simulink model "model_i3_c3_f2_equal_h2o"  (Simulink 8.4)
settings: Solver=ode3  StartTime=0.0  StopTime=1  FixedStep=0.0001  RelTol=1e-3
libraries: powerlib x28
settings Model: Creator=yh3wong  LastModifiedBy=yh3wong
settings DataIOCC: LimitDataPoints=off  SignalLoggingSaveFormat=Dataset  SaveOutput=off  SaveTime=off
settings OptimizationCC: ExpressionDepthLimit=128
settings DebuggingCC: UnderspecifiedInitializationDetection=Simplified  MergeDetectMultiDrivingBlocksExec=error  FcnCallInpInsideContextMsg=EnableAllAsError  UnconnectedInputMsg=none  UnconnectedOutputMsg=none  UnconnectedLineMsg=none  StateNameClashWarn=none
settings GRTTargetCC: CombineOutputUpdateFcns=on  GRTInterface=off

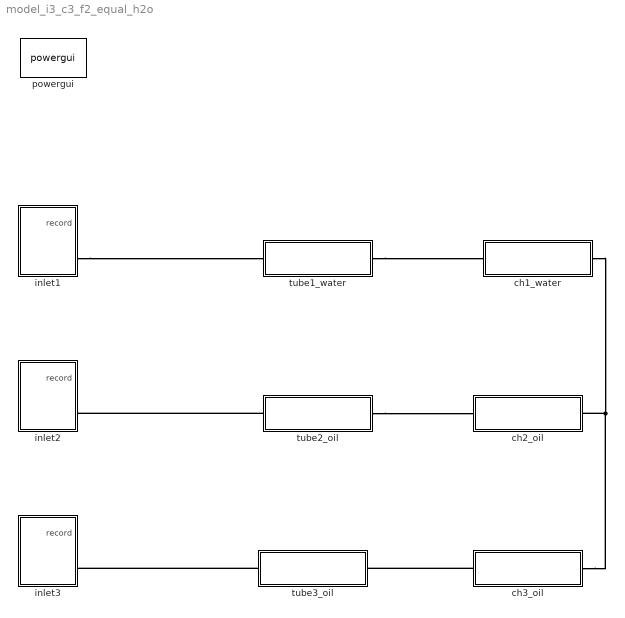
== system model_i3_c3_f2_equal_h2o ==
  ch1_water : Subsystem
  ch2_oil : Subsystem
  ch3_oil : Subsystem
  inlet1 : Subsystem
  inlet2 : Subsystem
  inlet3 : Subsystem
  powergui : powerlib/powergui  Priority=1  SimulationMode=Continuous  SolverType=Tustin/Backward Euler (TBE)  SampleTime=0.1  frequency=60  SPID=off  DisableSnubberDevices=off  DisableRonSwitches=off  DisableVfSwitches=off  SwTol=0  DisplayEquations=off  Interpol=off  methode=off  Ts=100  frequencyindice=0  Pbase=100e6  ErrMax=1e-4  Iterations=50  UnitsV=kV  UnitsW=MW  FunctionMessages=off  echomessages=off  HookPort=off  EnableUseOfTLC=off  x0status=blocks  RestoreLinks=warning  ResistiveCurrentMeasurement=off  Frange=[0:2:500]  Ylog=off  Xlog=on  ShowGrid=off  save=off  variable=ZData  structure=0  ZoomFFT=off  StartTime=0.0  cycles=1  DisplayStyle=1  fundamental=60  FreqAxis=off  MaxFrequency=1000  frequencyindicesteady=1  RmsSteady=1  display=off
  tube1_water : Subsystem
  tube2_oil : Subsystem
  tube3_oil : Subsystem
  connections:
  inlet1/RConn1 -- tube1_water/LConn1
  tube1_water/RConn1 -- ch1_water/LConn1
  tube2_oil/LConn1 -- inlet2/RConn1
  ch3_oil/LConn1 -- tube3_oil/RConn1
  tube3_oil/LConn1 -- inlet3/RConn1
  ch1_water/RConn1 -- ch3_oil/RConn1 -- ch2_oil/RConn1
  tube2_oil/RConn1 -- ch2_oil/LConn1

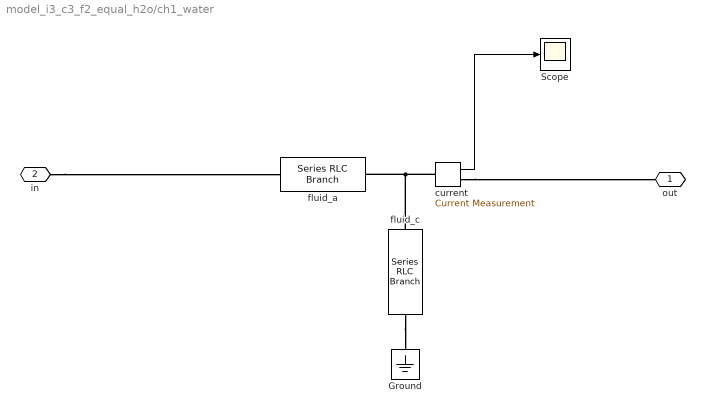
== system model_i3_c3_f2_equal_h2o/ch1_water ==
  Ground : powerlib/Elements/Ground  LConnTagsString=a
  Scope : Scope
      settings: ShowLegends=on  YMin=0  YMax=3e-11
  current : powerlib/Measurements/Current Measurement  PhasorSimulation=off  OutputType=Complex  PSBequivalent=0
  fluid_a : powerlib/Elements/Series RLC Branch  LConnTagsString=__new0  RConnTagsString=__new0  BranchType=RL  Resistance=0.000896  Inductance=7e-08  SetiL0=off  InitialCurrent=0  Capacitance=1e-6  Setx0=off  InitialVoltage=0  Measurements=None
  fluid_c : powerlib/Elements/Series RLC Branch  LConnTagsString=__new0  RConnTagsString=__new0  BranchType=C  Resistance=1  Inductance=1e-3  SetiL0=off  InitialCurrent=0  Capacitance=0.00032693  Setx0=off  InitialVoltage=0  Measurements=None
  out : PMIOPort  Port=1  Side=Right
  "in " : PMIOPort  Port=2  Side=Left
  wires:
  current/1 -> Scope/1
  connections:
  "in "/RConn1 -- fluid_a/LConn1
  fluid_c/RConn1 -- Ground/LConn1
  current/LConn1 -- fluid_a/RConn1 -- fluid_c/LConn1
  current/RConn1 -- out/RConn1

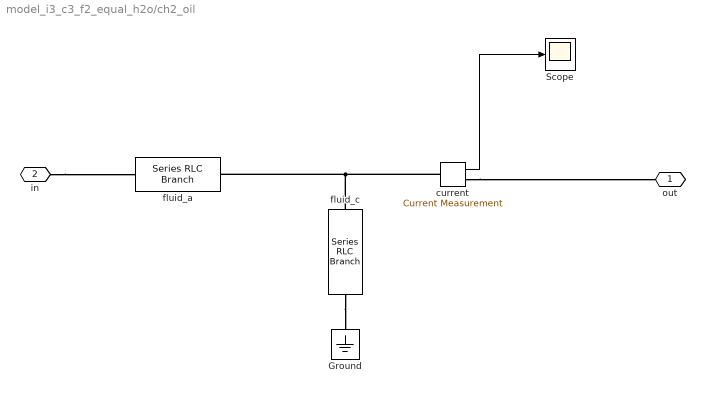
== system model_i3_c3_f2_equal_h2o/ch2_oil ==
  Ground : powerlib/Elements/Ground  LConnTagsString=a
  Scope : Scope
      settings: ShowLegends=on  YMin=0  YMax=3e-11
  current : powerlib/Measurements/Current Measurement  PhasorSimulation=off  OutputType=Complex  PSBequivalent=0
  fluid_a : powerlib/Elements/Series RLC Branch  LConnTagsString=__new0  RConnTagsString=__new0  BranchType=RL  Resistance=0.000896  Inductance=7e-08  SetiL0=off  InitialCurrent=0  Capacitance=1e-6  Setx0=off  InitialVoltage=0  Measurements=None
  fluid_c : powerlib/Elements/Series RLC Branch  LConnTagsString=__new0  RConnTagsString=__new0  BranchType=C  Resistance=1  Inductance=1e-3  SetiL0=off  InitialCurrent=0  Capacitance=0.00032693  Setx0=off  InitialVoltage=0  Measurements=None
  out : PMIOPort  Port=1  Side=Right
  "in " : PMIOPort  Port=2  Side=Left
  wires:
  current/1 -> Scope/1
  connections:
  "in "/RConn1 -- fluid_a/LConn1
  fluid_c/RConn1 -- Ground/LConn1
  current/LConn1 -- fluid_c/LConn1 -- fluid_a/RConn1
  current/RConn1 -- out/RConn1

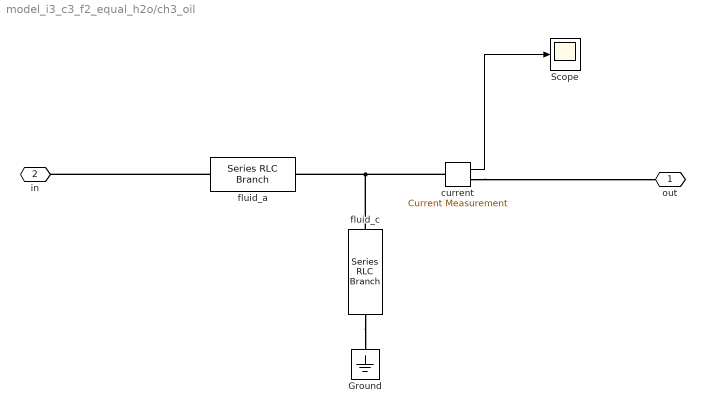
== system model_i3_c3_f2_equal_h2o/ch3_oil ==
  Ground : powerlib/Elements/Ground  LConnTagsString=a
  Scope : Scope
      settings: ShowLegends=on  YMin=0  YMax=3e-11
  current : powerlib/Measurements/Current Measurement  PhasorSimulation=off  OutputType=Complex  PSBequivalent=0
  fluid_a : powerlib/Elements/Series RLC Branch  LConnTagsString=__new0  RConnTagsString=__new0  BranchType=RL  Resistance=0.000896  Inductance=7e-08  SetiL0=off  InitialCurrent=0  Capacitance=1e-6  Setx0=off  InitialVoltage=0  Measurements=None
  fluid_c : powerlib/Elements/Series RLC Branch  LConnTagsString=__new0  RConnTagsString=__new0  BranchType=C  Resistance=1  Inductance=1e-3  SetiL0=off  InitialCurrent=0  Capacitance=0.00032693  Setx0=off  InitialVoltage=0  Measurements=None
  out : PMIOPort  Port=1  Side=Right
  "in " : PMIOPort  Port=2  Side=Left
  wires:
  current/1 -> Scope/1
  connections:
  fluid_c/RConn1 -- Ground/LConn1
  current/LConn1 -- fluid_c/LConn1 -- fluid_a/RConn1
  fluid_a/LConn1 -- "in "/RConn1
  current/RConn1 -- out/RConn1

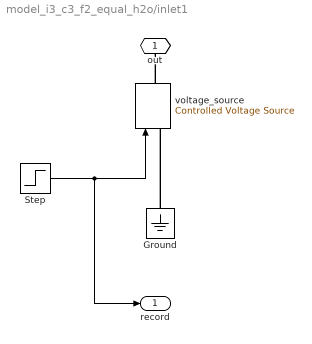
== system model_i3_c3_f2_equal_h2o/inlet1 ==
  Ground : powerlib/Elements/Ground  LConnTagsString=a
  Step : Step  Time=0.1  After=30000  SampleTime=0
  voltage_source : powerlib/Electrical Sources/Controlled Voltage Source  Initialize=on  Source_Type=DC  Amplitude=0  Phase=0  Frequency=0  Measurements=None
  out : PMIOPort  Port=1  Side=Right
  record : Outport
  wires:
  Step/1 -> record/1, voltage_source/1
  connections:
  Ground/LConn1 -- voltage_source/LConn1
  voltage_source/RConn1 -- out/RConn1

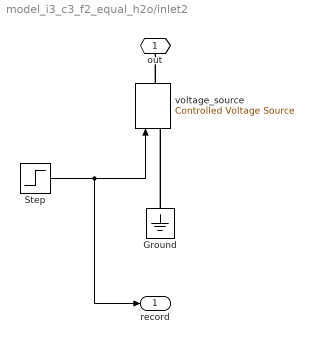
== system model_i3_c3_f2_equal_h2o/inlet2 ==
  Ground : powerlib/Elements/Ground  LConnTagsString=a
  Step : Step  Time=0.2  After=20000  SampleTime=0
  voltage_source : powerlib/Electrical Sources/Controlled Voltage Source  Initialize=on  Source_Type=DC  Amplitude=0  Phase=0  Frequency=0  Measurements=None
  out : PMIOPort  Port=1  Side=Right
  record : Outport
  wires:
  Step/1 -> record/1, voltage_source/1
  connections:
  Ground/LConn1 -- voltage_source/LConn1
  voltage_source/RConn1 -- out/RConn1

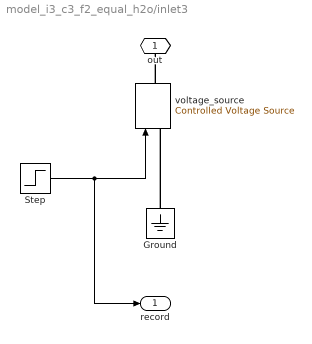
== system model_i3_c3_f2_equal_h2o/inlet3 ==
  Ground : powerlib/Elements/Ground  LConnTagsString=a
  Step : Step  Time=0.3  After=10000  SampleTime=0
  voltage_source : powerlib/Electrical Sources/Controlled Voltage Source  Initialize=on  Source_Type=DC  Amplitude=0  Phase=0  Frequency=0  Measurements=None
  out : PMIOPort  Port=1  Side=Right
  record : Outport
  wires:
  Step/1 -> record/1, voltage_source/1
  connections:
  Ground/LConn1 -- voltage_source/LConn1
  voltage_source/RConn1 -- out/RConn1

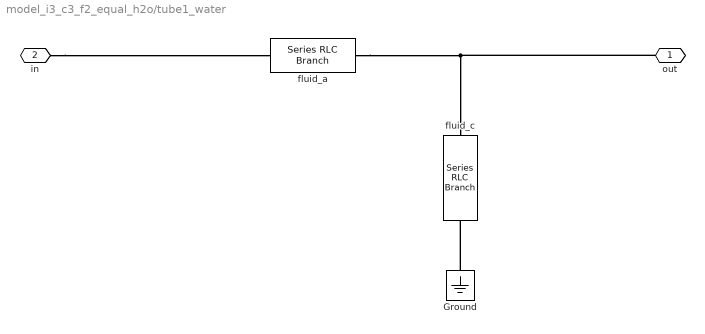
== system model_i3_c3_f2_equal_h2o/tube1_water ==
  Ground : powerlib/Elements/Ground  LConnTagsString=a
  fluid_a : powerlib/Elements/Series RLC Branch  LConnTagsString=__new0  RConnTagsString=__new0  BranchType=RL  Resistance=0.00027004  Inductance=4.9e-06  SetiL0=off  InitialCurrent=0  Capacitance=1e-6  Setx0=off  InitialVoltage=0  Measurements=None
  fluid_c : powerlib/Elements/Series RLC Branch  LConnTagsString=__new0  RConnTagsString=__new0  BranchType=C  Resistance=1  Inductance=1e-3  SetiL0=off  InitialCurrent=0  Capacitance=0.046394  Setx0=off  InitialVoltage=0  Measurements=None
  out : PMIOPort  Port=1  Side=Right
  "in " : PMIOPort  Port=2  Side=Left
  connections:
  "in "/RConn1 -- fluid_a/LConn1
  fluid_a/RConn1 -- out/RConn1 -- fluid_c/LConn1
  Ground/LConn1 -- fluid_c/RConn1

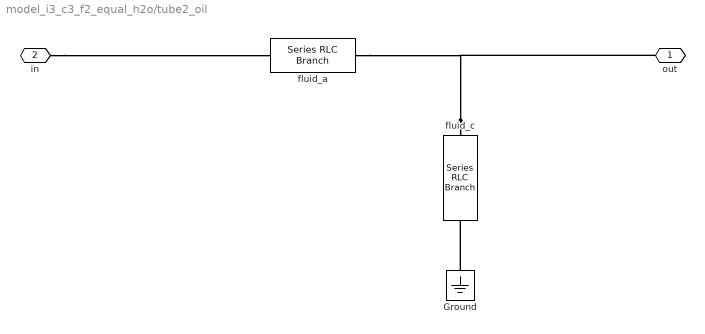
== system model_i3_c3_f2_equal_h2o/tube2_oil ==
  Ground : powerlib/Elements/Ground  LConnTagsString=a
  fluid_a : powerlib/Elements/Series RLC Branch  LConnTagsString=__new0  RConnTagsString=__new0  BranchType=RL  Resistance=0.00027004  Inductance=4.9e-06  SetiL0=off  InitialCurrent=0  Capacitance=1e-6  Setx0=off  InitialVoltage=0  Measurements=None
  fluid_c : powerlib/Elements/Series RLC Branch  LConnTagsString=__new0  RConnTagsString=__new0  BranchType=C  Resistance=1  Inductance=1e-3  SetiL0=off  InitialCurrent=0  Capacitance=0.046394  Setx0=off  InitialVoltage=0  Measurements=None
  out : PMIOPort  Port=1  Side=Right
  "in " : PMIOPort  Port=2  Side=Left
  connections:
  "in "/RConn1 -- fluid_a/LConn1
  fluid_c/LConn1 -- fluid_a/RConn1 -- out/RConn1
  Ground/LConn1 -- fluid_c/RConn1

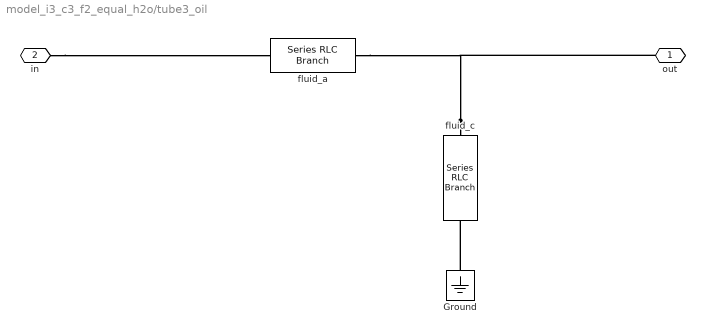
== system model_i3_c3_f2_equal_h2o/tube3_oil ==
  Ground : powerlib/Elements/Ground  LConnTagsString=a
  fluid_a : powerlib/Elements/Series RLC Branch  LConnTagsString=__new0  RConnTagsString=__new0  BranchType=RL  Resistance=0.00027004  Inductance=4.9e-06  SetiL0=off  InitialCurrent=0  Capacitance=1e-6  Setx0=off  InitialVoltage=0  Measurements=None
  fluid_c : powerlib/Elements/Series RLC Branch  LConnTagsString=__new0  RConnTagsString=__new0  BranchType=C  Resistance=1  Inductance=1e-3  SetiL0=off  InitialCurrent=0  Capacitance=0.046394  Setx0=off  InitialVoltage=0  Measurements=None
  out : PMIOPort  Port=1  Side=Right
  "in " : PMIOPort  Port=2  Side=Left
  connections:
  "in "/RConn1 -- fluid_a/LConn1
  fluid_c/LConn1 -- fluid_a/RConn1 -- out/RConn1
  Ground/LConn1 -- fluid_c/RConn1
